simulink model "lqr_int_sim"  (R2023b)
settings: Solver=FixedStepAuto  StartTime=0.0  StopTime=SIMTIME  FixedStep=SIMSTEP  RelTol=1e-3
values from neighbouring files (symbols this model uses):
  A = [z33,    eye(3) ... (first row only)    [lqr_int.m]
  B = [z33, inv(M)]'    [lqr_int.m]
  beta_c = deg2rad(1)    [lqr_int.m]
  bias = [1e4;1e3;0]    [lqr_int.m]
  bias_switch = -1    [lqr_int.m]
  Bv = [z33 z33 ... (first row only)    [lqr_int.m]
  C = [eye(3,6)]    [lqr_int.m]
  Ki = -K(:,end-n_augm+1:end)    [lqr_int.m]
  Klqr = K(:,1:n_states)    [lqr_int.m]
  ref = [2 1 deg2rad(1)]    [lqr_int.m]
  V_curr = 2    [lqr_int.m]
  V_wind = 0    [lqr_int.m]
  wave_ampl = [0, 0, 0]    [lqr_int.m]
  wave_length = [70 70 70]    [lqr_int.m]
  x0 = zeros(n_states, 1)    [lqr_int.m]
  x0int = zeros(n_augm ,1)    [lqr_int.m]
undefined symbols (not defined in the file or in its folder): ocean_coeff, wind_coeff
settings Model: Creator=X20  LastModifiedBy=Lorenzo-Desk
settings DataIOCC: ReturnWorkspaceOutputs=off

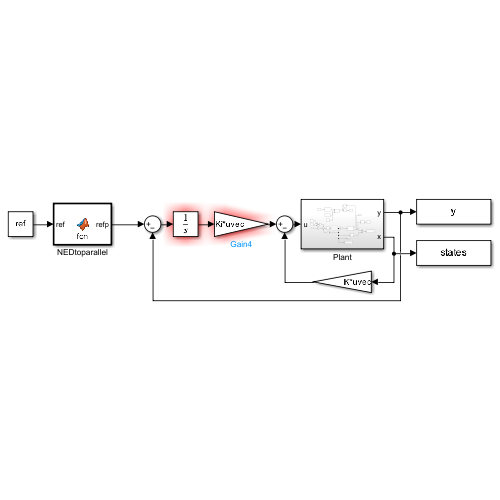
[thumbnail: Simulink's stored preview of the top-level diagram]
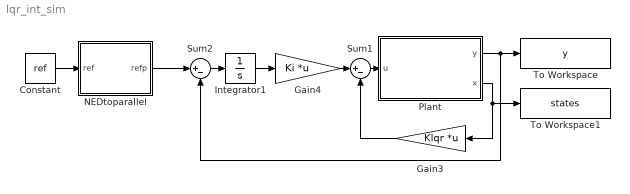
== system lqr_int_sim ==
  Constant : Constant  Value=ref
  Gain3 : Gain  Gain=Klqr  Multiplication=Matrix(K*u) (u vector)
  Gain4 : Gain  Gain=Ki  Multiplication=Matrix(K*u) (u vector)
  Integrator1 : Integrator  InitialCondition=x0int
  NEDtoparallel : MATLAB Function  TreatAsAtomicUnit=on
  Plant : Subsystem
  Sum1 : Sum  Inputs=|+-
  Sum2 : Sum  Inputs=|+-
  To Workspace : ToWorkspace  VariableName=y  SaveFormat=Timeseries  SampleTime=-1
  To Workspace1 : ToWorkspace  VariableName=states  SaveFormat=Timeseries  SampleTime=-1
  wires:
  Gain3/1 -> Sum1/2
  Gain4/1 -> Sum1/1
  Integrator1/1 -> Gain4/1
  Sum2/1 -> Integrator1/1
  Sum1/1 -> Plant/1(u)
  Plant/2(x) -> To Workspace1/1, Gain3/1
  Plant/1(y) -> Sum2/2, To Workspace/1
  Constant/1 -> NEDtoparallel/1(ref)
  NEDtoparallel/1(refp) -> Sum2/1

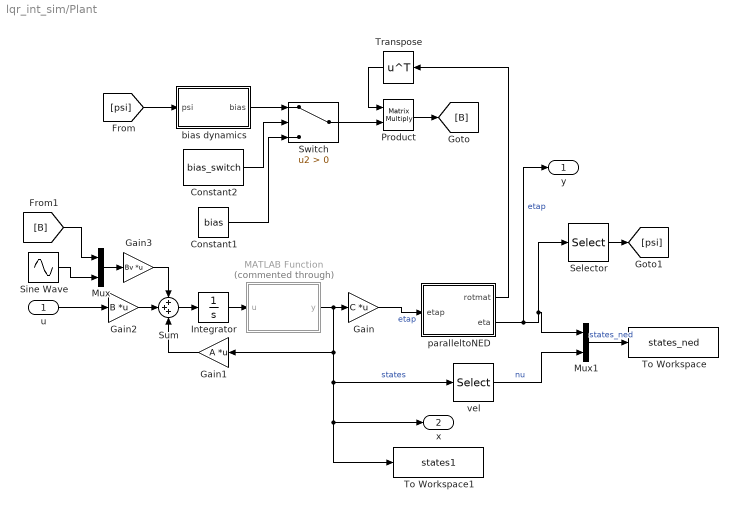
== system lqr_int_sim/Plant ==
  u : Inport
  Constant1 : Constant  Value=bias
  Constant2 : Constant  Value=bias_switch
  Gain : Gain  Gain=C  Multiplication=Matrix(K*u) (u vector)
  Gain1 : Gain  Gain=A  Multiplication=Matrix(K*u) (u vector)
  Gain2 : Gain  Gain=B  Multiplication=Matrix(K*u) (u vector)
  Gain3 : Gain  Gain=Bv  Multiplication=Matrix(K*u) (u vector)
  Integrator : Integrator  InitialCondition=x0
  MATLAB Function : MATLAB Function  Commented=through  TreatAsAtomicUnit=on
  Mux : Mux  Inputs=2
  Mux1 : Mux  Inputs=2
  Product : Product  Multiplication=Matrix(*)
  Selector : Selector  InputPortWidth=3  IndexOptions=Index vector (dialog)  Indices=[3]  OutputSizes=1
  Sine Wave : Sin  Amplitude=wave_ampl  Frequency=1./wave_length  SampleTime=0
  Sum : Sum  Inputs=+++
  Switch : Switch  Criteria=u2 > Threshold  SaturateOnIntegerOverflow=off  InputSameDT=off
  To Workspace : ToWorkspace  VariableName=states_ned  SaveFormat=Timeseries  SampleTime=-1
  To Workspace1 : ToWorkspace  VariableName=states1  SaveFormat=Timeseries  SampleTime=-1
  Transpose : Math  Operator=transpose
  bias dynamics : Subsystem
  paralleltoNED : MATLAB Function  TreatAsAtomicUnit=on
  vel : Selector  InputPortWidth=6  IndexOptions=Index vector (dialog)  Indices=[4 5 6]  OutputSizes=1
  y : Outport
  x : Outport  Port=2
  wires:
  Integrator/1 -> MATLAB Function/1(u)
  vel/1 -> Mux1/2  "nu"
  Sum/1 -> Integrator/1
  Mux/1 -> Gain3/1
  Gain2/1 -> Sum/2
  u/1 -> Gain2/1
  Gain/1 -> paralleltoNED/1(etap)  "etap"
  Selector/1 -> [psi]
  Sine Wave/1 -> Mux/2
  Constant1/1 -> Switch/3
  MATLAB Function/1(y) -> Gain/1, x/1, To Workspace1/1, vel/1, Gain1/1  "states"
  paralleltoNED/1(rotmat) -> Transpose/1
  Mux1/1 -> To Workspace/1  "states_ned"
  Gain1/1 -> Sum/3
  Gain3/1 -> Sum/1
  [psi] -> bias dynamics/1(psi)
  [B] -> Mux/1
  Transpose/1 -> Product/1
  bias dynamics/1(bias) -> Switch/1
  Product/1 -> [B]
  Switch/1 -> Product/2
  Constant2/1 -> Switch/2
  paralleltoNED/2(eta) -> y/1, Selector/1, Mux1/1  "etap"

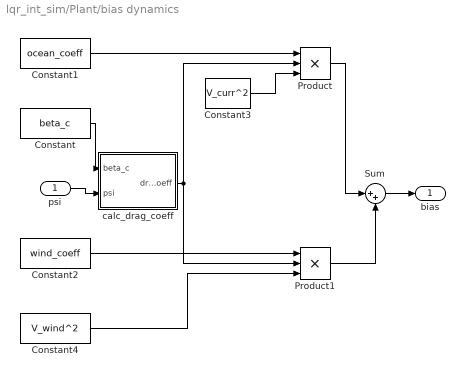
== system lqr_int_sim/Plant/bias dynamics ==
  psi : Inport
  Constant : Constant  Value=beta_c
  Constant1 : Constant  Value=ocean_coeff
  Constant2 : Constant  Value=wind_coeff
  Constant3 : Constant  Value=V_curr^2
  Constant4 : Constant  Value=V_wind^2
  Product : Product  Inputs=3
  Product1 : Product  Inputs=3
  Sum : Sum  Inputs=|++
  calc_drag_coeff : MATLAB Function  TreatAsAtomicUnit=on
  bias : Outport
  wires:
  psi/1 -> calc_drag_coeff/2(psi)
  Constant/1 -> calc_drag_coeff/1(beta_c)
  Constant4/1 -> Product1/3
  Product/1 -> Sum/1
  Product1/1 -> Sum/2
  Sum/1 -> bias/1
  Constant1/1 -> Product/1
  calc_drag_coeff/1(drag_coeff) -> Product1/2, Product/2
  Constant3/1 -> Product/3
  Constant2/1 -> Product1/1

== matlab function lqr_int_sim/Plant/paralleltoNED ==
  data: rotmat output; etap input; eta output
function [rotmat, eta] = fcn(etap)
    psip = etap(3);
    rotmat = [cos(psip), -sin(psip), 0; 
              sin(psip),  cos(psip), 0;
                      0,          0, 1];
    eta = rotmat*etap;
end

== matlab function lqr_int_sim/Plant/MATLAB Function ==
  data: u input; y output
function y = fcn(u)
    u(3) = wrapTo2Pi(u(3)) - pi;
    y = u;
end

== matlab function lqr_int_sim/NEDtoparallel ==
  data: refp output; ref input
function refp  = fcn(ref)
    psi = ref(3);
    rotmat = [cos(psi), -sin(psi), 0; 
              sin(psi),  cos(psi), 0;
                      0,          0, 1];
    refp = rotmat'*ref;
end

== matlab function lqr_int_sim/Plant/bias dynamics/calc_drag_coeff ==
  data: beta_c input; drag_coeff output; psi input
function drag_coeff = fcn(beta_c, psi)
    angle_of_attack = psi-beta_c-pi;
    cx = 0.7;
    cy = 0.8; 
    cn = 0.15;
    Cx = -cx*cos(angle_of_attack);
    Cy = cy*sin(angle_of_attack);
    Cn = cn*sin(2*angle_of_attack);
    drag_coeff = [Cx, Cy, Cn]';
end
